simulink model "Channelizer_DFT_testbench"  (R2021a)
settings: Solver=VariableStepAuto  StartTime=0.0  StopTime=N*2  RelTol=1e-3
InitFcn:
  | N=16;
  | sample_size=4;
undefined symbols (not defined in the file or in its folder): S, vsva2197, xcvc1902
libraries: aieBasic x17, aieUtilities x8, dspxfrm3 x2, vmcUtilities x1
settings Model: Creator=robg  LastModifiedBy=robg
settings DataIOCC: SaveFormat=Array  SaveOutput=off  SignalLogging=off  DSMLogging=off  SaveTime=off

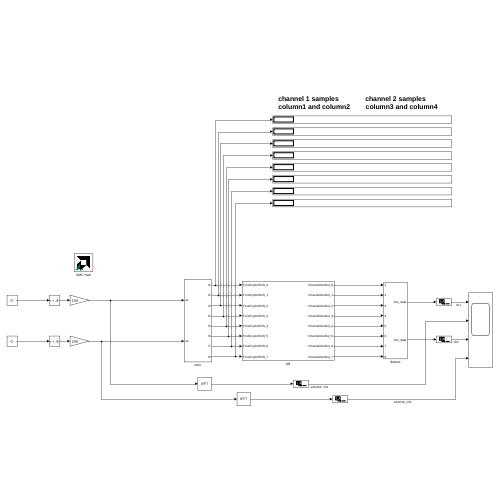
[thumbnail: Simulink's stored preview of the top-level diagram]
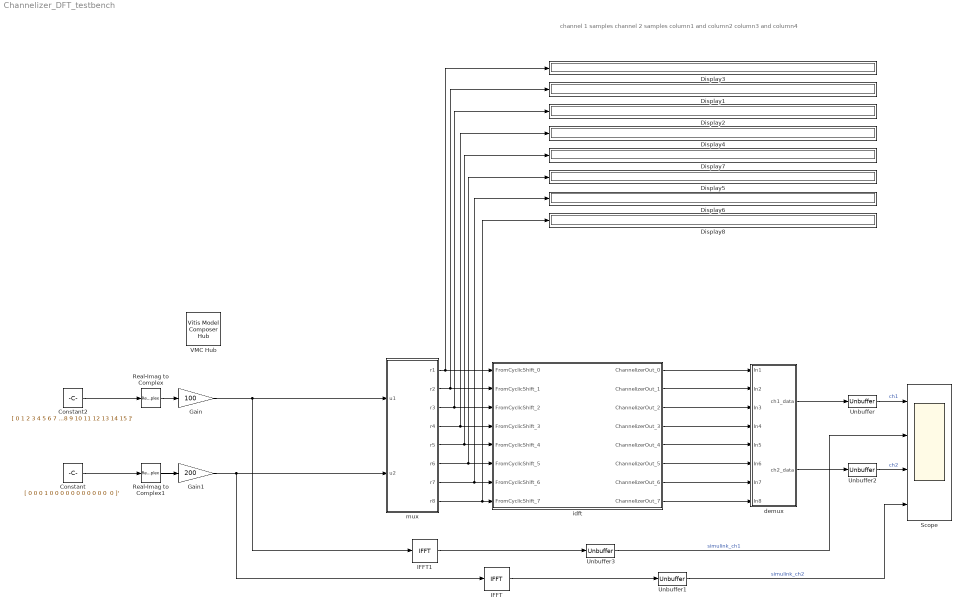
== system Channelizer_DFT_testbench ==
  note: channel 1 samples channel 2 samples
      | column1 and column2 column3 and column4
  Constant : Constant  Value="[ 0 0 0 1 0 0 0 0 0 0 0 0 0 0 0  0 ]'"  VectorParams1D=off  OutDataTypeStr=int16  SampleTime=N
  Constant2 : Constant  Value=[ 0 1 2 3 4 5 6 7 8 9 10 11 12 13 14 15 ]'  VectorParams1D=off  OutDataTypeStr=int16  SampleTime=N
  Display{1..8} (8 alike) : Display
  Gain : Gain  Gain=100  OutDataTypeStr=int16
  Gain1 : Gain  Gain=200  OutDataTypeStr=int16
  IFFT : dspxfrm3/IFFT  FFTImplementation=Auto  CompMethod=Table lookup  TableOpt=NEW  TableOptActive=Speed  BitRevOrder=off  cs_in=off  Normalize=off  InheritFFTLength=on  FFTLength=64  WrapInput=on  mode=Complex  outSamplingMode=Sample based  roundingMode=Floor  overflowMode=off  firstCoeffDataTypeStr=Inherit: Same word length as input  firstCoeffLastDataTypeStr=Inherit: Same word length as input  prodOutputMode=Binary point scaling  prodOutputWordLength=32  prodOutputFracLength=0  prodOutputDataTypeStr=fixdt(1,32,0)  prodOutputLastDataTypeStr=fixdt(1,32,0)  outputMode=Binary point scaling  outputWordLength=16  outputFracLength=0  outputDataTypeStr=fixdt(1,16,0)  outputMin=[]  outputMax=[]  outputLastDataTypeStr=fixdt(1,16,0)
  IFFT1 : dspxfrm3/IFFT  FFTImplementation=Auto  CompMethod=Table lookup  TableOpt=NEW  TableOptActive=Speed  BitRevOrder=off  cs_in=off  Normalize=off  InheritFFTLength=on  FFTLength=64  WrapInput=on  mode=Complex  outSamplingMode=Sample based  roundingMode=Floor  overflowMode=off  firstCoeffDataTypeStr=Inherit: Same word length as input  firstCoeffLastDataTypeStr=Inherit: Same word length as input  prodOutputMode=Binary point scaling  prodOutputWordLength=32  prodOutputFracLength=0  prodOutputDataTypeStr=fixdt(1,32,0)  prodOutputLastDataTypeStr=fixdt(1,32,0)  outputMode=Binary point scaling  outputWordLength=16  outputFracLength=0  outputDataTypeStr=fixdt(1,16,0)  outputMin=[]  outputMax=[]  outputLastDataTypeStr=fixdt(1,16,0)
  Real-Imag to Complex : RealImagToComplex  Input=Real
  Real-Imag to Complex1 : RealImagToComplex  Input=Real
  Scope : Scope  NumInputPorts=4
  Unbuffer{,1..3} (4 alike) : Unbuffer
  VMC Hub : vmcUtilities/Vitis Model Composer Hub  Tag=genX  CodeGeneration=off  TargetDirectory=./code  ExportType=AI Engines  IpVendor=xilinx.com  IpLibrary=hls  IpVersion=1.0  IpHWLanguage=Verilog  AieCompilerOptions={}  AieSimulatorOptions={}  CreateTestbench=off  TestbenchStackSize=10  RunAieSim=off  AieSimTimeout=50000  RunAieSimProfiling=off  LaunchVitisAnalyzer=off  PlotOutput=off  RunX86Sim=off  X86SimTimeout=10  GenHwImage=off  PlatformType=Not Specified  HwSystemType=Baremetal  HwValidationTarget=hw  ProjDevice=Versal VCK190 Evaluation Platform with New SD Level Shifter (xcvc1902-vsva2197-2MP-e-S)  ProjDevicePart=xcvc1902-vsva2197-2MP-e-S  SamplePeriod=-1  ClockFrequency=200  DataPathParallelism=1  xilinxfamily=versalaicore  part=xcvc1902  speed=-2MP-e-S  package=vsva2197  directory=./netlist  testbench=off  incr_netlist=off  synthesis_tool=Vivado  clock_wrapper=Clock Enables  dbl_ovrd=According to Block Masks  dcm_input_clock_period=10  sysclk_period=10  simulink_period=1  eval_field=0  LogFileName=''  NThreads=4
  demux : Subsystem
  idft : Subsystem
  mux : Subsystem
  wires:
  idft/2(ChannelizerOut_1) -> demux/2(In2)
  idft/3(ChannelizerOut_2) -> demux/3(In3)
  idft/1(ChannelizerOut_0) -> demux/1(In1)
  idft/5(ChannelizerOut_4) -> demux/5(In5)
  idft/7(ChannelizerOut_6) -> demux/7(In7)
  demux/1(ch1_data) -> Unbuffer/1
  idft/6(ChannelizerOut_5) -> demux/6(In6)
  idft/8(ChannelizerOut_7) -> demux/8(In8)
  Unbuffer1/1 -> Scope/4  "simulink_ch2"
  Unbuffer/1 -> Scope/1  "ch1"
  IFFT/1 -> Unbuffer1/1
  idft/4(ChannelizerOut_3) -> demux/4(In4)
  demux/2(ch2_data) -> Unbuffer2/1
  Unbuffer2/1 -> Scope/3  "ch2"
  IFFT1/1 -> Unbuffer3/1
  Unbuffer3/1 -> Scope/2  "simulink_ch1"
  Real-Imag to Complex/1 -> Gain/1
  Real-Imag to Complex1/1 -> Gain1/1
  Gain/1 -> mux/1(u1), IFFT1/1
  Gain1/1 -> mux/2(u2), IFFT/1
  Constant/1 -> Real-Imag to Complex1/1
  Constant2/1 -> Real-Imag to Complex/1
  mux/8(r8) -> Display8/1, idft/8(FromCyclicShift_7)
  mux/3(r3) -> Display2/1, idft/3(FromCyclicShift_2)
  mux/7(r7) -> Display6/1, idft/7(FromCyclicShift_6)
  mux/2(r2) -> Display1/1, idft/2(FromCyclicShift_1)
  mux/5(r5) -> Display7/1, idft/5(FromCyclicShift_4)
  mux/6(r6) -> Display5/1, idft/6(FromCyclicShift_5)
  mux/4(r4) -> Display4/1, idft/4(FromCyclicShift_3)
  mux/1(r1) -> idft/1(FromCyclicShift_0), Display3/1

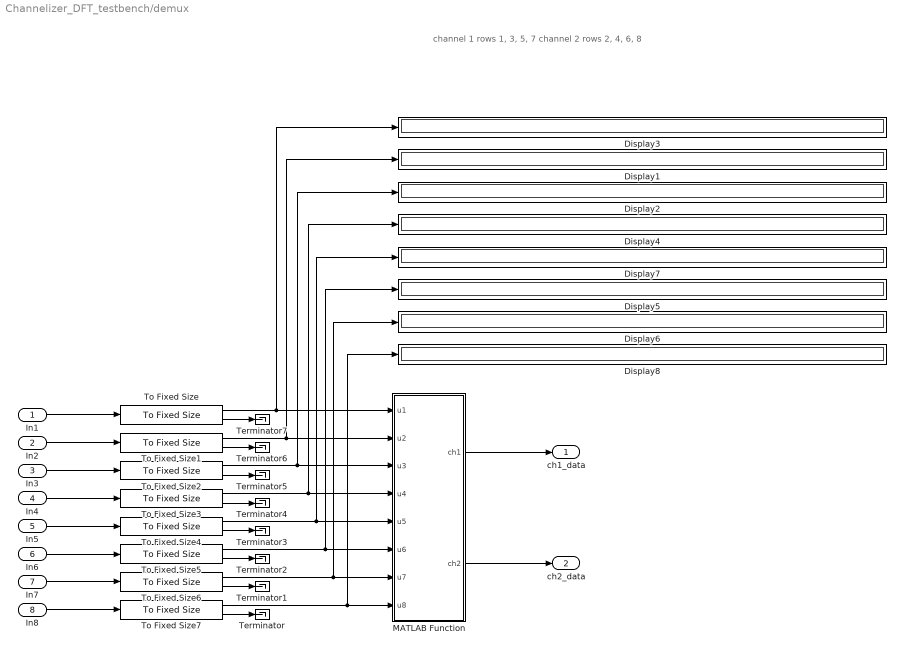
== system Channelizer_DFT_testbench/demux ==
  note: channel 1 rows 1, 3, 5, 7
      | channel 2 rows 2, 4, 6, 8
  In1 : Inport
  In2 : Inport  Port=2
  In3 : Inport  Port=3
  In4 : Inport  Port=4
  In5 : Inport  Port=5
  In6 : Inport  Port=6
  In7 : Inport  Port=7
  In8 : Inport  Port=8
  Display{1..8} (8 alike) : Display
  MATLAB Function : MATLAB Function  TreatAsAtomicUnit=on
  Terminator{,1..7} (8 alike) : Terminator
  To Fixed Size{,1..7} (8 alike) : aieUtilities/To Fixed Size  OutputSize=Inherit: Same as input  CopyMethod=Buffer samples to form output  HasStatusOutput=on  Mode=Produce a valid output signal
  ch1_data : Outport
  ch2_data : Outport  Port=2
  wires:
  In1/1 -> To Fixed Size/1
  In2/1 -> To Fixed Size1/1
  In3/1 -> To Fixed Size2/1
  In4/1 -> To Fixed Size3/1
  In5/1 -> To Fixed Size4/1
  In6/1 -> To Fixed Size5/1
  In7/1 -> To Fixed Size6/1
  In8/1 -> To Fixed Size7/1
  MATLAB Function/1(ch1) -> ch1_data/1
  MATLAB Function/2(ch2) -> ch2_data/1
  To Fixed Size/1 -> Display3/1, MATLAB Function/1(u1)
  To Fixed Size1/1 -> Display1/1, MATLAB Function/2(u2)
  To Fixed Size2/1 -> Display2/1, MATLAB Function/3(u3)
  To Fixed Size3/1 -> Display4/1, MATLAB Function/4(u4)
  To Fixed Size4/1 -> Display7/1, MATLAB Function/5(u5)
  To Fixed Size5/1 -> Display5/1, MATLAB Function/6(u6)
  To Fixed Size6/1 -> Display6/1, MATLAB Function/7(u7)
  To Fixed Size7/1 -> Display8/1, MATLAB Function/8(u8)
  To Fixed Size7/2 -> Terminator/1
  To Fixed Size6/2 -> Terminator1/1
  To Fixed Size5/2 -> Terminator2/1
  To Fixed Size4/2 -> Terminator3/1
  To Fixed Size3/2 -> Terminator4/1
  To Fixed Size2/2 -> Terminator5/1
  To Fixed Size1/2 -> Terminator6/1
  To Fixed Size/2 -> Terminator7/1

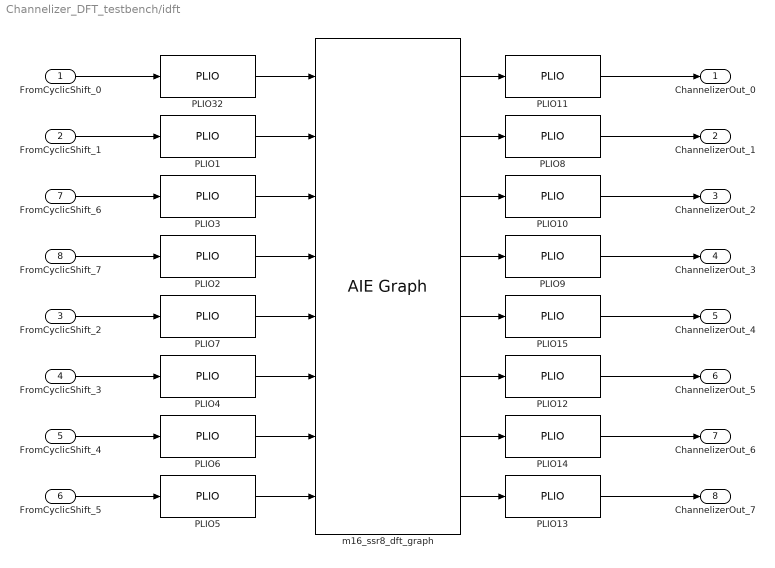
== system Channelizer_DFT_testbench/idft ==
  FromCyclicShift_0 : Inport
  FromCyclicShift_1 : Inport  Port=2
  FromCyclicShift_2 : Inport  Port=3
  FromCyclicShift_3 : Inport  Port=4
  FromCyclicShift_4 : Inport  Port=5
  FromCyclicShift_5 : Inport  Port=6
  FromCyclicShift_6 : Inport  Port=7
  FromCyclicShift_7 : Inport  Port=8
  PLIO{1..15,32} (16 alike) : aieBasic/PLIO  PlioWidth=64  PlioFreqSpec=on  PlioFreq=625  ColLocation=0  channel=0  blockJsonConstraints=[]  deprecateConstraints=0
  m16_ssr8_dft_graph : aieBasic/AIE Graph  PortAttributesTable={ 'Input', 'sig_i[0]', 'stream', 'cint16', '', '', ''; 'Input', 'sig_i[1]', 'stream', 'cint16', '', '', ''; 'Input', 'sig_i[6]', 'stream', 'cint16', '', '', ''; 'Input', 'sig_i[7]', 'stream', 'cint16', '', '', ''; 'Input', 'sig_i[2]', 'stream', 'cint16', '', '', ''; 'Input', 'sig_i[3]', 'stream', 'cint16', '', '', ''; 'Input', 'sig_i[4]', 'stream', 'cint16', '', '', ''; 'Input', 'sig_i[5]', 'stream', 'cint16', '', '', ''; 'Output', 'sig_o[0]', 'stream', 'cint16', '', '', '4'; 'Output', 'sig_o[1]', 'stream', 'cint16', '', '', '4'; 'Output', 'sig_o[2]', 'stream', 'cint16', '', '', '4'; 'Output', 'sig_o[3]', 'stream', 'cint16', '', '', '4'; 'Output', 'sig_o[4]', 'stream', 'cint16', '', '', '4'; 'Output', 'sig_o[5]', 'stream', 'cint16', '', '', '4'; 'Output', 'sig_o[6]', 'stream', 'cint16', '', '', '4'; 'Output', 'sig_o[7]', 'stream', 'cint16', '', '', '4' }  PortAttributesEnablement={'off', 'on', 'off', 'off', 'off', 'off', 'off';'off', 'on', 'off', 'off', 'off', 'off', 'off';'off', 'on', 'off', 'off', 'off', 'off', 'off';'off', 'on', 'off', 'off', 'off', 'off', 'off';'off', 'on', 'off', 'off', 'off', 'off', 'off';'off', 'on', 'off', 'off', 'off', 'off', 'off';'off', 'on', 'off', 'off', 'off', 'off', 'off';'off', 'on', 'off', 'off', 'off', 'off', 'off';'off', 'on', 'off', 'off', 'off', 'off', 'on';'off', 'on', 'off', 'off', 'off', 'off', 'on';'off', 'on', 'off', 'off', 'off', 'off', 'on';'off', 'on', 'off', 'off', 'off', 'off', 'on';'off', 'on', 'off', 'off', 'off', 'off', 'on';'off', 'on', 'off', 'off', 'off', 'off', 'on';'off', 'on', 'off', 'off', 'off', 'off', 'on';'off', 'on', 'off', 'off', 'off', 'off', 'on'}  SampleTime=-1  ClassDeclTypeOptions=C[1 1]@t24@class m16_ssr8_dft_graph  ClassDecl=<empty>  ClassTemplateParams={}  ClassTemplateParamsEnables={}  ClassPortParams={}  ClassCtorDeclTypeOptions=C[1 1]@t7@<empty>  ClassCtorDecl=<empty>  ClassCtorParams={}  GraphAllAttrs=|  PortArgDecls={'in stream cint16 in1'; 'in stream cint16 in2'; 'in stream cint16 in3'; 'in stream cint16 in4'; 'in stream cint16 in5'; 'in stream cint16 in6'; 'in stream cint16 in7'; 'in stream cint16 in8'; 'out stream cint16 out1'; 'out stream cint16 out2'; 'out stream cint16 out3'; 'out stream cint16 out4'; 'out stream cint16 out5'; 'out stream cint16 out6'; 'out stream cint16 out7'; 'out stream cint16 out8'}  PortGraphPortNames={'sig_i[0]'; 'sig_i[1]'; 'sig_i[6]'; 'sig_i[7]'; 'sig_i[2]'; 'sig_i[3]'; 'sig_i[4]'; 'sig_i[5]'; 'sig_o[0]'; 'sig_o[1]'; 'sig_o[2]'; 'sig_o[3]'; 'sig_o[4]'; 'sig_o[5]'; 'sig_o[6]'; 'sig_o[7]'}  PortTypes={'stream'; 'stream'; 'stream'; 'stream'; 'stream'; 'stream'; 'stream'; 'stream'; 'stream'; 'stream'; 'stream'; 'stream'; 'stream'; 'stream'; 'stream'; 'stream'}  PortDataTypes={'cint16'; 'cint16'; 'cint16'; 'cint16'; 'cint16'; 'cint16'; 'cint16'; 'cint16'; 'cint16'; 'cint16'; 'cint16'; 'cint16'; 'cint16'; 'cint16'; 'cint16'; 'cint16'}  PortSizes={0.000000000000000000e+00; 0.000000000000000000e+00; 0.000000000000000000e+00; 0.000000000000000000e+00; 0.000000000000000000e+00; 0.000000000000000000e+00; 0.000000000000000000e+00; 0.000000000000000000e+00; 0.000000000000000000e+00; 0.000000000000000000e+00; 0.000000000000000000e+00; 0.000000000000000000e+00; 0.000000000000000000e+00; 0.000000000000000000e+00; 0.000000000000000000e+00; 0.000000000000000000e+00}  PortSynchronicities={'auto'; 'auto'; 'auto'; 'auto'; 'auto'; 'auto'; 'auto'; 'auto'; 'auto'; 'auto'; 'auto'; 'auto'; 'auto'; 'auto'; 'auto'; 'auto'}  PortSignalSizes={0.000000000000000000e+00; 0.000000000000000000e+00; 0.000000000000000000e+00; 0.000000000000000000e+00; 0.000000000000000000e+00; 0.000000000000000000e+00; 0.000000000000000000e+00; 0.000000000000000000e+00; 4.000000000000000000e+00; 4.000000000000000000e+00; 4.000000000000000000e+00; 4.000000000000000000e+00; 4.000000000000000000e+00; 4.000000000000000000e+00; 4.000000000000000000e+00; 4.000000000000000000e+00}  SimLibPath=''  ClassIndex=1  ClassCtorIndex=0  ClassTabVisible=off  FunctionTabVisible=on  DelayDrawLabels=off  GraphFileSelect=Header file (*.h)  GraphHeaderFile=m16_ssr8_dft_graph.h  GraphClassName=m16_ssr8_dft_graph  GraphName=m16_ssr8_dft_graph  GraphHeaderFiles={'./aie/dft_1xN_widget_graph.h'; './aie/m16_ssr8_dft_graph.h'}  GraphSourceFile=./model_composer_work/xmc_aie_lib/8d40d72d/mygraph.cpp  GraphSearchPaths={}  GraphPreProcOptions={}  blockJsonConstraints=[]  deprecateConstraints=0
      | s[12;12;9;9;19;14;21;23;21;23;24;21;15;17;12;24;26;26;26;27;28;9;21;23;23;23;24;25;14;19;19;29]@FunctionNameDeclFileNamePortNamesPortTypesPortSerializedTypesPortDirectionsPortWindowSizeEnablesPortWindowMarginEnablesPortBufferSizeEnablesPortBufferMarginEnablesPortSynchronicityEnablesPortSignalSizeEnablesPortBufferSizesPortBufferMarginsFunctionDeclFunctionTemplateSpecKindFunctionTemplateParamNamesFunctionTemplateParamKindsFunctionTemplateParamTypesFunctionTemplateParamValuesFunctionTemplateParamEnablesClassDeclClassTemplateSpecKindClassTemplateParamNamesClassTemplateParamKindsClassTemplateParamTypesClassTemplateParamValuesClassTemplateParamEnablesClassCtorDeclsClassCtorParamNamesClassCtorParamTypesClassCtorParamSerializedTypes[1 1]@C[32 1]@nt30@../../aie/m16_ssr8_dft_graph.hC[2 1]@t5@sig_it5@sig_oC[2 1]@t48@std::array< adf::port< adf::direction::in >, 8 >t49@std::array< adf::port< adf::direction::out >, 8 >C[2 1]@t64@{Tstd::array{2{t{Tadf::port{1{t{Sadf::direction::in}}}}}{t{}8}}}t65@{Tstd::array{2{t{Tadf::port{1{t{Sadf::direction::out}}}}}{t{}8}}}C[2 1]@t5@inputt5@inputC[2 1]@l0@l0@C[2 1]@l0@l0@C[2 1]@l0@l0@C[2 1]@l0@l0@C[2 1]@l1@l1@C[2 1]@l0@l0@C[2 1]@nnC[2 1]@nnt139@void m16_ssr8_dft_graph::
      | (std::array< adf::port< adf::direction::in >, 8 > sig_i, std::array< adf::port< adf::direction::out >, 8 > sig_o)ne[0 1]@e[0 1]@e[0 1]@e[0 1]@e[0 1]@t25@class m16_ssr8_dft_graph;t4@nonee[0 1]@e[0 1]@e[0 1]@e[0 1]@e[0 1]@e[0 1]@e[0 1]@e[0 1]@e[0 1]@
  ChannelizerOut_0 : Outport
  ChannelizerOut_1 : Outport  Port=2
  ChannelizerOut_2 : Outport  Port=3
  ChannelizerOut_3 : Outport  Port=4
  ChannelizerOut_4 : Outport  Port=5
  ChannelizerOut_5 : Outport  Port=6
  ChannelizerOut_6 : Outport  Port=7
  ChannelizerOut_7 : Outport  Port=8
  wires:
  PLIO15/1 -> ChannelizerOut_4/1
  PLIO7/1 -> m16_ssr8_dft_graph/5
  FromCyclicShift_5/1 -> PLIO5/1
  m16_ssr8_dft_graph/1 -> PLIO11/1
  FromCyclicShift_7/1 -> PLIO2/1
  FromCyclicShift_4/1 -> PLIO6/1
  PLIO2/1 -> m16_ssr8_dft_graph/4
  PLIO3/1 -> m16_ssr8_dft_graph/3
  PLIO9/1 -> ChannelizerOut_3/1
  FromCyclicShift_0/1 -> PLIO32/1
  FromCyclicShift_3/1 -> PLIO4/1
  PLIO11/1 -> ChannelizerOut_0/1
  PLIO10/1 -> ChannelizerOut_2/1
  PLIO32/1 -> m16_ssr8_dft_graph/1
  PLIO8/1 -> ChannelizerOut_1/1
  PLIO4/1 -> m16_ssr8_dft_graph/6
  FromCyclicShift_1/1 -> PLIO1/1
  PLIO6/1 -> m16_ssr8_dft_graph/7
  FromCyclicShift_2/1 -> PLIO7/1
  PLIO5/1 -> m16_ssr8_dft_graph/8
  PLIO1/1 -> m16_ssr8_dft_graph/2
  PLIO13/1 -> ChannelizerOut_7/1
  PLIO14/1 -> ChannelizerOut_6/1
  FromCyclicShift_6/1 -> PLIO3/1
  PLIO12/1 -> ChannelizerOut_5/1
  m16_ssr8_dft_graph/2 -> PLIO8/1
  m16_ssr8_dft_graph/3 -> PLIO10/1
  m16_ssr8_dft_graph/4 -> PLIO9/1
  m16_ssr8_dft_graph/5 -> PLIO15/1
  m16_ssr8_dft_graph/6 -> PLIO12/1
  m16_ssr8_dft_graph/7 -> PLIO14/1
  m16_ssr8_dft_graph/8 -> PLIO13/1

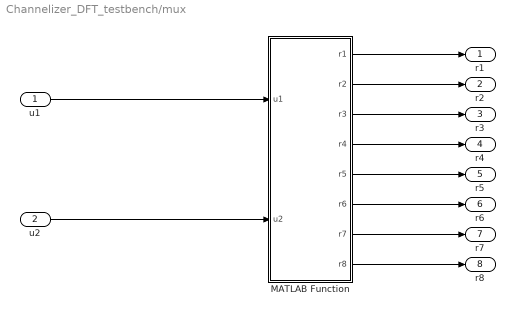
== system Channelizer_DFT_testbench/mux ==
  u1 : Inport
  u2 : Inport  Port=2
  MATLAB Function : MATLAB Function  TreatAsAtomicUnit=on
  r1 : Outport
  r2 : Outport  Port=2
  r3 : Outport  Port=3
  r4 : Outport  Port=4
  r5 : Outport  Port=5
  r6 : Outport  Port=6
  r7 : Outport  Port=7
  r8 : Outport  Port=8
  wires:
  MATLAB Function/6(r6) -> r6/1
  u1/1 -> MATLAB Function/1(u1)
  MATLAB Function/7(r7) -> r7/1
  MATLAB Function/8(r8) -> r8/1
  MATLAB Function/3(r3) -> r3/1
  MATLAB Function/5(r5) -> r5/1
  u2/1 -> MATLAB Function/2(u2)
  MATLAB Function/2(r2) -> r2/1
  MATLAB Function/4(r4) -> r4/1
  MATLAB Function/1(r1) -> r1/1

== matlab function Channelizer_DFT_testbench/demux/MATLAB Function ==
  data: u1 input; ch1 output; u2 input; u3 input; u4 input; u5 input; u6 input; u7 input; u8 input; ch2 output
function [ch1,ch2] = fcn(u1, u2, u3, u4, u5, u6, u7, u8)
%#codegen

ch1 = [ u1 ; u3 ; u5 ; u7 ];

ch2 = [ u2 ; u4 ; u6 ; u8 ];

== matlab function Channelizer_DFT_testbench/mux/MATLAB Function ==
  data: u1 input; r1 output; r2 output; r3 output; r4 output; r5 output; r6 output; r7 output; r8 output; u2 input
function [r1,r2,r3,r4,r5,r6,r7,r8]  = fcn(u1, u2)

r1 = [ u1(1,1) ; u1(2,1) ; u2(1,1) ; u2(2,1) ];
r2 = [ u1(3,1) ; u1(4,1) ; u2(3,1) ; u2(4,1) ];
r3 = [ u1(5,1) ; u1(6,1) ; u2(5,1) ; u2(6,1) ];
r4 = [ u1(7,1) ; u1(8,1) ; u2(7,1) ; u2(8,1) ];
r5 = [ u1(9,1) ; u1(10,1) ; u2(9,1) ; u2(10,1) ];
r6 = [ u1(11,1) ; u1(12,1) ; u2(11,1) ; u2(12,1) ];
r7 = [ u1(13,1) ; u1(14,1) ; u2(13,1) ; u2(14,1) ];
r8 = [ u1(15,1) ; u1(16,1) ; u2(15,1) ; u2(16,1) ];
